simulink model "mDataStoreBlocksVariants"  (R2013b)
settings: Solver=FixedStepDiscrete  StartTime=0.0  StopTime=10.0  RelTol=1e-3
PreLoadFcn:
  | VSS_NONLINEAR_CONTROLLER=Simulink.Variant('VSS_MODE==1')
  | VSS_SECOND_ORDER_CONTROLLER=Simulink.Variant('VSS_MODE==2')
  | 
  | VSS_MODE=1
Description:
  | Variant Subsystems
  | 
  | This model illustrates Simulink(R) variant subsystems. Variant subsystems let
  | you provide multiple implementations to a subsystem where only one
  | implementation is active during simulation. You can programmatically swap out
  | the active implementation and replace it with one of the other implementations
  | without modifying the model.
settings Model: FPTRunName=Active  Creator=The MathWorks Inc.  LastModifiedBy=hungdang
settings DataIOCC: SignalLoggingSaveFormat=ModelDataLogs
settings OptimizationCC: InlineParams=on  ExpressionDepthLimit=2147483647
settings DebuggingCC: FcnCallInpInsideContextMsg=UseLocalSettings  StateNameClashWarn=warning
settings RTWCC: ProcessScript=grt_make_rtw_hook
settings GRTTargetCC: CombineOutputUpdateFcns=off  GRTInterface=on

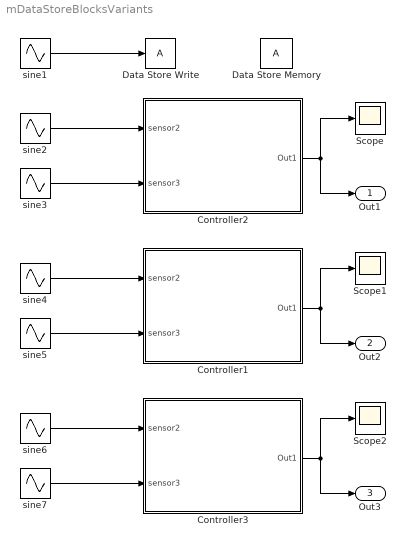
== system mDataStoreBlocksVariants ==
  Controller1 : Subsystem  Variant=on
  Controller2 : Subsystem  Variant=on
  Controller3 : Subsystem  Variant=on
  Data Store Memory : DataStoreMemory  ReadBeforeWriteMsg=warning  WriteAfterWriteMsg=warning  WriteAfterReadMsg=warning
  Data Store Write : DataStoreWrite  SampleTime=0.01
  Scope : Scope
  Scope1 : Scope
  Scope2 : Scope
      settings: SaveName=ScopeData2
  sine1 : Sin  Amplitude=.1  Frequency=pi/3  SampleTime=.01
  sine2 : Sin  Amplitude=2  SampleTime=.01
  sine3 : Sin  Amplitude=.3  Frequency=pi/6  SampleTime=.01
  sine4 : Sin  Amplitude=2  SampleTime=.01
  sine5 : Sin  Amplitude=.3  Frequency=pi/6  SampleTime=.01
  sine6 : Sin  Amplitude=2  SampleTime=.01
  sine7 : Sin  Amplitude=.3  Frequency=pi/6  SampleTime=.01
  Out1 : Outport
  Out2 : Outport  Port=2
  Out3 : Outport  Port=3
  wires:
  sine2/1 -> Controller2/1(sensor2)
  sine3/1 -> Controller2/2(sensor3)
  Controller2/1(Out1) -> Scope/1, Out1/1
  sine1/1 -> Data Store Write/1
  sine4/1 -> Controller1/1(sensor2)
  sine5/1 -> Controller1/2(sensor3)
  Controller1/1(Out1) -> Scope1/1, Out2/1
  sine6/1 -> Controller3/1(sensor2)
  sine7/1 -> Controller3/2(sensor3)
  Controller3/1(Out1) -> Scope2/1, Out3/1

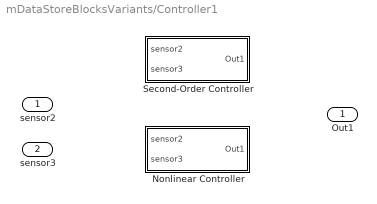
== system mDataStoreBlocksVariants/Controller1 ==
  sensor2 : Inport
  sensor3 : Inport  Port=2
  Nonlinear Controller : Subsystem  VariantControl=VSS_NONLINEAR_CONTROLLER
  Second-Order Controller : Subsystem  VariantControl=VSS_SECOND_ORDER_CONTROLLER
  Out1 : Outport

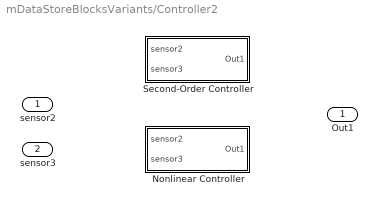
== system mDataStoreBlocksVariants/Controller2 ==
  sensor2 : Inport
  sensor3 : Inport  Port=2
  Nonlinear Controller : Subsystem  VariantControl=VSS_NONLINEAR_CONTROLLER
  Second-Order Controller : Subsystem  VariantControl=VSS_SECOND_ORDER_CONTROLLER
  Out1 : Outport

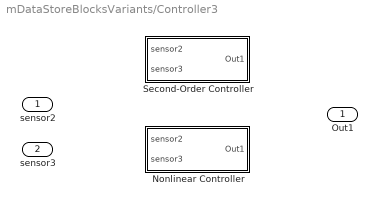
== system mDataStoreBlocksVariants/Controller3 ==
  sensor2 : Inport
  sensor3 : Inport  Port=2
  Nonlinear Controller : Subsystem  VariantControl=VSS_NONLINEAR_CONTROLLER
  Second-Order Controller : Subsystem  VariantControl=VSS_SECOND_ORDER_CONTROLLER
  Out1 : Outport

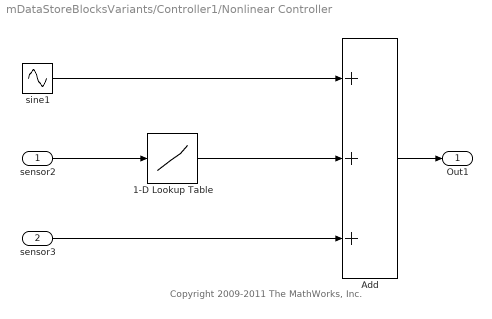
== system mDataStoreBlocksVariants/Controller1/Nonlinear Controller ==
  note: Copyright 2009-2011 The MathWorks, Inc.
  sensor2 : Inport
  sensor3 : Inport  Port=2
  1-D Lookup Table : Lookup_n-D  NumberOfTableDimensions=1  BreakpointsForDimension1=[-5:5]  Table=tanh([-5:5])  InputSameDT=on
  Add : Sum  Inputs=+++  SampleTime=.01
  sine1 : Sin  Amplitude=.1  Frequency=pi/3  SampleTime=.01
  Out1 : Outport
  wires:
  sensor2/1 -> 1-D Lookup Table/1
  1-D Lookup Table/1 -> Add/2
  sensor3/1 -> Add/3
  sine1/1 -> Add/1
  Add/1 -> Out1/1

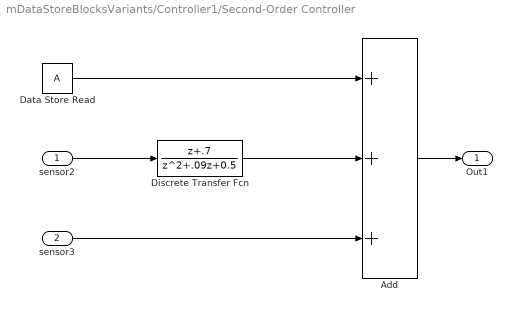
== system mDataStoreBlocksVariants/Controller1/Second-Order Controller ==
  sensor2 : Inport
  sensor3 : Inport  Port=2
  Add : Sum  Inputs=+++
  Data Store Read : DataStoreRead  SampleTime=0.01
  Discrete Transfer Fcn : DiscreteTransferFcn  Numerator=[1 .7]  Denominator=[1 .09 0.5]  SampleTime=.01
  Out1 : Outport
  wires:
  sensor2/1 -> Discrete Transfer Fcn/1
  Discrete Transfer Fcn/1 -> Add/2
  sensor3/1 -> Add/3
  Data Store Read/1 -> Add/1
  Add/1 -> Out1/1

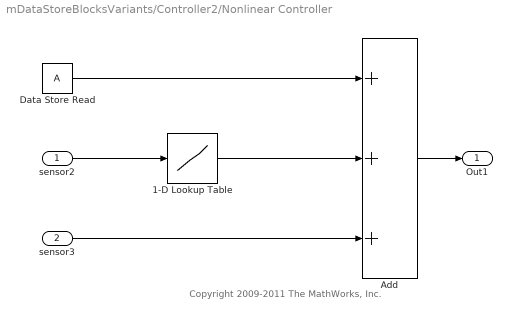
== system mDataStoreBlocksVariants/Controller2/Nonlinear Controller ==
  note: Copyright 2009-2011 The MathWorks, Inc.
  sensor2 : Inport
  sensor3 : Inport  Port=2
  1-D Lookup Table : Lookup_n-D  NumberOfTableDimensions=1  BreakpointsForDimension1=[-5:5]  Table=tanh([-5:5])  InputSameDT=on
  Add : Sum  Inputs=+++  SampleTime=.01
  Data Store Read : DataStoreRead  SampleTime=0.01
  Out1 : Outport
  wires:
  sensor2/1 -> 1-D Lookup Table/1
  1-D Lookup Table/1 -> Add/2
  sensor3/1 -> Add/3
  Data Store Read/1 -> Add/1
  Add/1 -> Out1/1

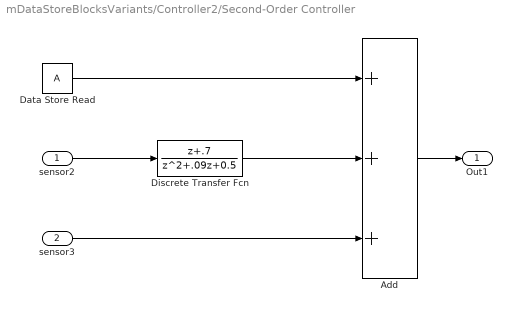
== system mDataStoreBlocksVariants/Controller2/Second-Order Controller ==
  sensor2 : Inport
  sensor3 : Inport  Port=2
  Add : Sum  Inputs=+++
  Data Store Read : DataStoreRead  SampleTime=0.01
  Discrete Transfer Fcn : DiscreteTransferFcn  Numerator=[1 .7]  Denominator=[1 .09 0.5]  SampleTime=.01
  Out1 : Outport
  wires:
  sensor2/1 -> Discrete Transfer Fcn/1
  Discrete Transfer Fcn/1 -> Add/2
  sensor3/1 -> Add/3
  Data Store Read/1 -> Add/1
  Add/1 -> Out1/1

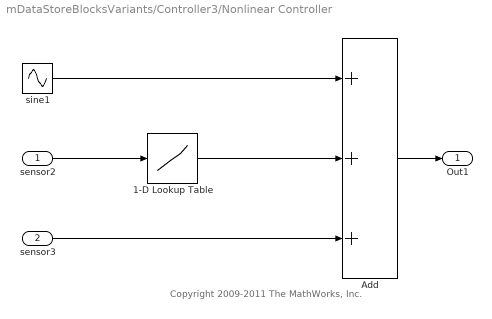
== system mDataStoreBlocksVariants/Controller3/Nonlinear Controller ==
  note: Copyright 2009-2011 The MathWorks, Inc.
  sensor2 : Inport
  sensor3 : Inport  Port=2
  1-D Lookup Table : Lookup_n-D  NumberOfTableDimensions=1  BreakpointsForDimension1=[-5:5]  Table=tanh([-5:5])  InputSameDT=on
  Add : Sum  Inputs=+++  SampleTime=.01
  sine1 : Sin  Amplitude=.1  Frequency=pi/3  SampleTime=.01
  Out1 : Outport
  wires:
  sensor2/1 -> 1-D Lookup Table/1
  1-D Lookup Table/1 -> Add/2
  sensor3/1 -> Add/3
  sine1/1 -> Add/1
  Add/1 -> Out1/1

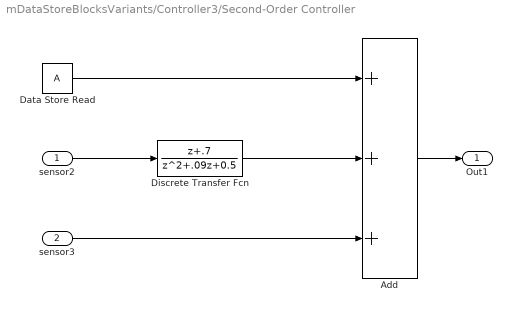
== system mDataStoreBlocksVariants/Controller3/Second-Order Controller ==
  sensor2 : Inport
  sensor3 : Inport  Port=2
  Add : Sum  Inputs=+++
  Data Store Read : DataStoreRead  SampleTime=0.01
  Discrete Transfer Fcn : DiscreteTransferFcn  Numerator=[1 .7]  Denominator=[1 .09 0.5]  SampleTime=.01
  Out1 : Outport
  wires:
  sensor2/1 -> Discrete Transfer Fcn/1
  Discrete Transfer Fcn/1 -> Add/2
  sensor3/1 -> Add/3
  Data Store Read/1 -> Add/1
  Add/1 -> Out1/1
